simulink subsystem "Reefscape_Auto_sub"  (R2023b)
settings: Solver=VariableStepAuto  StartTime=0.0  StopTime=10.0  RelTol=1e-3
undefined symbols (not defined in the file): All_Paths_Num_Poses, All_Paths_Ref_Poses, AT_Steering_Error_Angle_Gain_P, AT_Steering_Speed_Max, AT_Translation_Control_Gain_Relative, AT_Translation_Speed_Max_Relative, Auto_Starting_Position
libraries: simulink x3
settings Model: Creator=ander  LastModifiedBy=ander

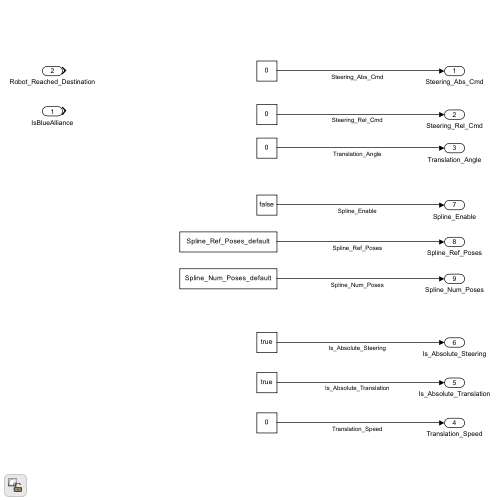
[thumbnail: Simulink's stored preview of the top-level diagram]
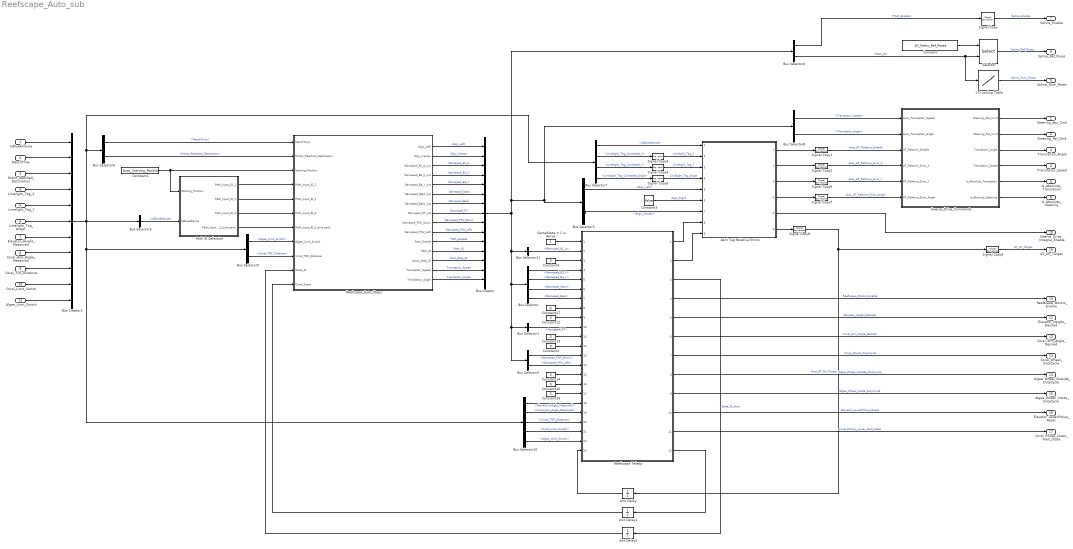
== system Reefscape_Auto_sub ==
  IsBlueAlliance : Inport
  MatchTime : Inport  Port=2
  Robot_Reached_Destination : Inport  Port=3
  Limelight_Tag_X : Inport  Port=4
  Limelight_Tag_Y : Inport  Port=5
  Limelight_Tag_Angle : Inport  Port=6
  Elevator_Height_Measured : Inport  Port=7
  Coral_Arm_Angle_Measured : Inport  Port=8
  Coral_TOF_Distance : Inport  Port=9
  Coral_Limit_Switch : Inport  Port=10
  Algae_Limit_Switch : Inport  Port=11
  1-D Lookup Table : Lookup_n-D  NumberOfTableDimensions=1  BreakpointsSpecification=Even spacing  BreakpointsForDimension1=[-5:5]  Table=All_Paths_Num_Poses  InterpMethod=Flat  InternalRulePriority=Speed  OutDataTypeStr=double  RndMeth=Simplest
  April Tag Relative Errors : Subsystem  ReferencedSubsystem=April_Tag_Relative_Errors
  Bus Creator : BusCreator  Inputs=15
  Bus Creator2 : BusCreator  Inputs=11
  Bus Selector : BusSelector  OutputSignals=Gamepad_B3_X,Gamepad_B4_Y,Gamepad_Start,Gamepad_Back
  Bus Selector1 : BusSelector  OutputSignals=Gamepad_RT
  Bus Selector10 : BusSelector  OutputSignals=Elevator_Height_Measured,Coral_Arm_Angle_Measured,Coral_TOF_Distance,Coral_Limit_Switch,Algae_Limit_Switch
  Bus Selector11 : BusSelector  OutputSignals=Gamepad_B1_A
  Bus Selector2 : BusSelector  OutputSignals=Gamepad_POV_Down,Gamepad_POV_Left
  Bus Selector3 : BusSelector  OutputSignals=Align_Left,Align_Center
  Bus Selector4 : BusSelector  OutputSignals=Path_Enable,Path_ID
  Bus Selector5 : BusSelector  OutputSignals=IsBlueAlliance
  Bus Selector6 : BusSelector  OutputSignals=MatchTime,Robot_Reached_Destination
  Bus Selector7 : BusSelector  OutputSignals=IsBlueAlliance,Limelight_Tag_Corrected_X,Limelight_Tag_Corrected_Y,Limelight_Tag_Corrected_Angle
  Bus Selector8 : BusSelector  OutputSignals=Translation_Speed,Translation_Angle
  Bus Selector9 : BusSelector  OutputSignals=Algae_Limit_Switch,Coral_TOF_Distance
  Constant : Constant  Value=All_Paths_Ref_Poses
  Constant1 : Constant  Value=Auto_Starting_Position  OutDataTypeStr=double
  Constant{2,4,12..14,17} (6 alike) : Constant  Value=0  OutDataTypeStr=boolean
  Constant15 : Constant  Value=0  OutDataTypeStr=double
  Constant16 : Constant  Value=0  OutDataTypeStr=double
  Constant3 : Constant  Value=false  OutDataTypeStr=boolean
  GameState = 1 is Autos : Constant  OutDataTypeStr=uint8
  Path ID Selection : Subsystem
  Reefscape Teleop : Subsystem  ReferencedSubsystem=Reefscape_Teleop_sub
  Reefscape_Auto_Steps : Stateflow chart  TreatAsAtomicUnit=on
      settings: PortSchema="{\"entries\":[{\"content\":{\"sides\":[{\"content\":{\"connectorIds\":[\"In1\",\"In2\",\"In3\",\"In4\",\"In5\",\"In6\",\"In7\",\"In8\",\"In9\",\"In11\",\"In10\"]},\"type\":\"ConnectorPlacement.EquallySpacedRectSide\",\"uuid\":\"b68629cc-4697-4054-9cba-8a9d44fa304a\"},{\"content\":{\"connectorIds\":[\"Out1\",\"Out2\",\"Out14\",\"Out15\",\"Out3\",\"Out4\",\"Out5\",\"Out6\",\"Out7\",\"Out8\",\"Out9\",\"Out10\",\"Out11\",\"Out12\",\"Out13\"],\"side\":\"RIGHT\"},\"type\":\"ConnectorPlacement.EquallySpacedRectSide\",\"uuid\":\"e5ec4660-532e-44af-95ac-1c70b52239a5\"},{\"content\":{\"side\":\"TOP\"},\"type\":\"ConnectorPlacement.EquallySpacedRectSide\",\"uuid\":\"c81c735c-b6d1-4ece-b5d5-793d4c0e4420\"}]},\"type\":\"ConnectorPlacement.EquallySpacedConnector\",\"uuid\":\"b2f2970a-f1c8-496a-85fd-16c79425c6c1\"}],\"packageUris\":[\"http://schema.mathworks.com/mf0/Connector/R2020b\"],\"version\":\"1.0\"}"
  Selector : Selector  NumberOfDimensions=3  InputPortWidth=3  IndexOptions=Select all,Select all,Index vector (port)  Indices=[1 3],1,1  OutputSizes=1,1,1
  Signal Copy{,1..9} (10 alike) : SignalConversion  OverrideOpt=off
  Swerve_Drive_Commands : Subsystem
  Unit Delay : UnitDelay  SampleTime=-1  HasFrameUpgradeWarning=on
  Unit Delay1 : UnitDelay  SampleTime=-1  HasFrameUpgradeWarning=on
  Unit Delay2 : UnitDelay  SampleTime=-1  HasFrameUpgradeWarning=on
  Steering_Abs_Cmd : Outport
  Steering_Rel_Cmd : Outport  Port=2
  Translation_Angle : Outport  Port=3
  Translation_Speed : Outport  Port=4
  Is_Absolute_Translation : Outport  Port=5
  Is_Absolute_Steering : Outport  Port=6
  Spline_Enable : Outport  Port=7
  Spline_Ref_Poses : Outport  Port=8
  Spline_Num_Poses : Outport  Port=9
  Reefscape_Motors_Enable : Outport  Port=10
  Elevator_Height_Desired : Outport  Port=11
  Coral_Arm_Angle_Desired : Outport  Port=12
  Coral_Wheel_DutyCycle : Outport  Port=13
  Algae_Wheel_Outside_DutyCycle : Outport  Port=14
  Algae_Wheel_Inside_DutyCycle : Outport  Port=15
  Elevator_LowerPickup_Reset : Outport  Port=16
  Coral_Pickup_Lower_Wait_State : Outport  Port=17
  Swerve_Drive_Integral_Enable : Outport  Port=18
  AT_On_Target : Outport  Port=19
  wires:
  Constant3/1 -> April Tag Relative Errors/6  "Align_Right"
  Unit Delay/1 -> Reefscape Teleop/23
  Bus Selector10/5 -> Reefscape Teleop/22  "<Algae_Limit_Switch>"
  Bus Selector10/4 -> Reefscape Teleop/21  "<Coral_Limit_Switch>"
  Bus Selector10/3 -> Reefscape Teleop/20  "<Coral_TOF_Distance>"
  Bus Selector10/2 -> Reefscape Teleop/19  "<Coral_Arm_Angle_Measured>"
  Bus Selector10/1 -> Reefscape Teleop/18  "<Elevator_Height_Measured>"
  Constant16/1 -> Reefscape Teleop/17
  Constant15/1 -> Reefscape Teleop/16
  Constant14/1 -> Reefscape Teleop/15
  Bus Selector2/2 -> Reefscape Teleop/14  "<Gamepad_POV_Left>"
  Bus Selector2/1 -> Reefscape Teleop/13  "<Gamepad_POV_Down>"
  Constant2/1 -> Reefscape Teleop/12
  1-D Lookup Table/1 -> Spline_Num_Poses/1  "Spline_Num_Poses"
  Signal Copy/1 -> Spline_Enable/1  "Spline_Enable"
  Selector/1 -> Spline_Ref_Poses/1  "Spline_Ref_Poses"
  Constant/1 -> Selector/1
  Bus Selector6/2 -> Reefscape_Auto_Steps/2(Robot_Reached_Destination)  "<Robot_Reached_Destination>"
  Constant1/1 -> Reefscape_Auto_Steps/3(Starting_Position), Path ID Selection/1(Starting_Position)
  Path ID Selection/3(Path_Input_ID_3) -> Reefscape_Auto_Steps/6(Path_Input_ID_3)
  Bus Selector5/1 -> Path ID Selection/2(IsBlueAlliance)  "<IsBlueAlliance>"
  Path ID Selection/1(Path_Input_ID_1) -> Reefscape_Auto_Steps/4(Path_Input_ID_1)
  Path ID Selection/2(Path_Input_ID_2) -> Reefscape_Auto_Steps/5(Path_Input_ID_2)
  Signal Copy5/1 -> April Tag Relative Errors/4  "Limelight_Tag_Angle"
  Signal Copy4/1 -> April Tag Relative Errors/3  "Limelight_Tag_Y"
  Signal Copy3/1 -> April Tag Relative Errors/2  "Limelight_Tag_X"
  Reefscape Teleop/1 -> April Tag Relative Errors/8
  Reefscape Teleop/2 -> April Tag Relative Errors/9
  April Tag Relative Errors/6 -> Signal Copy8/1
  Bus Creator/1 -> Bus Selector11/1, Bus Selector/1, Bus Selector1/1, Bus Selector2/1, Bus Selector4/1, Bus Selector8/1, Bus Selector3/1
  Bus Selector3/1 -> April Tag Relative Errors/5  "<Align_Left>"
  Bus Selector3/2 -> April Tag Relative Errors/7  "<Align_Center>"
  Reefscape_Auto_Steps/1(Align_Left) -> Bus Creator/1  "Align_Left"
  Reefscape_Auto_Steps/2(Align_Center) -> Bus Creator/2  "Align_Center"
  Unit Delay1/1 -> Reefscape_Auto_Steps/10(Coral_Score)
  Bus Selector4/1 -> Signal Copy/1  "<Path_Enable>"
  Bus Selector4/2 -> Selector/2, 1-D Lookup Table/1  "<Path_ID>"
  IsBlueAlliance/1 -> Bus Creator2/1
  Bus Creator2/1 -> Bus Selector10/1, Bus Selector9/1, Bus Selector5/1, Bus Selector6/1, Bus Selector7/1
  Bus Selector7/1 -> April Tag Relative Errors/1  "<IsBlueAlliance>"
  Bus Selector9/1 -> Reefscape_Auto_Steps/8(Algae_Limit_Switch)  "<Algae_Limit_Switch>"
  April Tag Relative Errors/2 -> Signal Copy2/1
  April Tag Relative Errors/1 -> Signal Copy1/1
  April Tag Relative Errors/3 -> Signal Copy6/1
  April Tag Relative Errors/4 -> Signal Copy7/1
  April Tag Relative Errors/5 -> Swerve_Drive_Integral_Enable/1
  Swerve_Drive_Commands/1(Steering_Abs_Cmd) -> Steering_Abs_Cmd/1
  Swerve_Drive_Commands/2(Steering_Rel_Cmd) -> Steering_Rel_Cmd/1
  Swerve_Drive_Commands/3(Translation_Angle) -> Translation_Angle/1
  Swerve_Drive_Commands/4(Translation_Speed) -> Translation_Speed/1
  Swerve_Drive_Commands/5(Is_Absolute_Translation) -> Is_Absolute_Translation/1
  Swerve_Drive_Commands/6(Is_Absolute_Steering) -> Is_Absolute_Steering/1
  Bus Selector8/2 -> Swerve_Drive_Commands/2(Auto_Translation_Angle)  "<Translation_Angle>"
  Bus Selector8/1 -> Swerve_Drive_Commands/1(Auto_Translation_Speed)  "<Translation_Speed>"
  Bus Selector7/2 -> Signal Copy3/1  "<Limelight_Tag_Corrected_X>"
  Bus Selector7/3 -> Signal Copy4/1  "<Limelight_Tag_Corrected_Y>"
  Bus Selector7/4 -> Signal Copy5/1  "<Limelight_Tag_Corrected_Angle>"
  Reefscape Teleop/4 -> Reefscape_Motors_Enable/1  "Reefscape_Motors_Enable"
  Reefscape Teleop/5 -> Elevator_Height_Desired/1  "Elevator_Height_Desired"
  Reefscape Teleop/6 -> Coral_Arm_Angle_Desired/1  "Coral_Arm_Angle_Desired"
  Reefscape Teleop/7 -> Coral_Wheel_DutyCycle/1  "Coral_Wheel_DutyCycle"
  Reefscape Teleop/8 -> Algae_Wheel_Outside_DutyCycle/1  "Algae_Wheel_Outside_DutyCycle"
  Reefscape Teleop/9 -> Algae_Wheel_Inside_DutyCycle/1  "Algae_Wheel_Inside_DutyCycle"
  Reefscape Teleop/10 -> Elevator_LowerPickup_Reset/1  "Elevator_LowerPickup_Reset"
  Reefscape Teleop/11 -> Coral_Pickup_Lower_Wait_State/1  "Coral_Pickup_Lower_Wait_State"
  GameState = 1 is Autos/1 -> Reefscape Teleop/1
  Reefscape Teleop/12 -> Unit Delay1/1
  Algae_Limit_Switch/1 -> Bus Creator2/11
  Coral_Limit_Switch/1 -> Bus Creator2/10
  Coral_TOF_Distance/1 -> Bus Creator2/9
  Coral_Arm_Angle_Measured/1 -> Bus Creator2/8
  Elevator_Height_Measured/1 -> Bus Creator2/7
  Limelight_Tag_Angle/1 -> Bus Creator2/6
  Limelight_Tag_Y/1 -> Bus Creator2/5
  Limelight_Tag_X/1 -> Bus Creator2/4
  Robot_Reached_Destination/1 -> Bus Creator2/3
  Signal Copy1/1 -> Swerve_Drive_Commands/3(AT_Relative_Enable)  "Auto_AT_Relative_Enable"
  Signal Copy2/1 -> Swerve_Drive_Commands/4(AT_Relative_Error_X)  "Auto_AT_Relative_Error_X"
  Signal Copy6/1 -> Swerve_Drive_Commands/5(AT_Relative_Error_Y)  "Auto_AT_Relative_Error_Y"
  Signal Copy7/1 -> Swerve_Drive_Commands/6(AT_Relative_Error_Angle)  "Auto_AT_Relative_Error_Angle"
  Signal Copy8/1 -> Unit Delay/1, Signal Copy9/1  "Auto_AT_On_Target"
  Signal Copy9/1 -> AT_On_Target/1  "AT_On_Target"
  Bus Selector9/2 -> Reefscape_Auto_Steps/9(Coral_TOF_Distance)  "<Coral_TOF_Distance>"
  Constant4/1 -> Reefscape Teleop/3
  Bus Selector/2 -> Reefscape Teleop/5  "<Gamepad_B4_Y>"
  Bus Selector/3 -> Reefscape Teleop/6  "<Gamepad_Start>"
  Bus Selector/4 -> Reefscape Teleop/7  "<Gamepad_Back>"
  Constant17/1 -> Reefscape Teleop/8
  Constant13/1 -> Reefscape Teleop/11
  Reefscape Teleop/3 -> Unit Delay2/1  "State_ID_Auto"
  Path ID Selection/4(Path_Input_ID_2_end_early) -> Reefscape_Auto_Steps/7(Path_Input_ID_2_end_early)
  Constant12/1 -> Reefscape Teleop/9
  Bus Selector1/1 -> Reefscape Teleop/10  "<Gamepad_RT>"
  Unit Delay2/1 -> Reefscape_Auto_Steps/11(State_ID)
  Reefscape_Auto_Steps/14(Gamepad_B1_A_out) -> Bus Creator/3  "Gamepad_B1_A"
  Reefscape_Auto_Steps/3(Gamepad_B4_Y_out) -> Bus Creator/5  "Gamepad_B4_Y"
  Reefscape_Auto_Steps/4(Gamepad_Start_out) -> Bus Creator/6  "Gamepad_Start"
  Reefscape_Auto_Steps/5(Gamepad_Back_out) -> Bus Creator/7  "Gamepad_Back"
  Reefscape_Auto_Steps/6(Gamepad_RT_out) -> Bus Creator/8  "Gamepad_RT"
  Reefscape_Auto_Steps/7(Gamepad_POV_Down) -> Bus Creator/9  "Gamepad_POV_Down"
  Reefscape_Auto_Steps/8(Gamepad_POV_Left) -> Bus Creator/10  "Gamepad_POV_Left"
  Reefscape_Auto_Steps/9(Path_Enable) -> Bus Creator/11  "Path_Enable"
  Reefscape_Auto_Steps/10(Path_ID) -> Bus Creator/12  "Path_ID"
  Reefscape_Auto_Steps/11(Autos_Step_ID) -> Bus Creator/13  "Auto_Step_ID"
  Reefscape_Auto_Steps/12(Translation_Speed) -> Bus Creator/14  "Translation_Speed"
  Reefscape_Auto_Steps/13(Translation_Angle) -> Bus Creator/15  "Translation_Angle"
  Bus Selector11/1 -> Reefscape Teleop/2  "<Gamepad_B1_A>"
  Reefscape_Auto_Steps/15(Gamepad_B3_X_out) -> Bus Creator/4  "Gamepad_B3_X"
  Bus Selector/1 -> Reefscape Teleop/4  "<Gamepad_B3_X>"
  MatchTime/1 -> Bus Creator2/2
  Bus Selector6/1 -> Reefscape_Auto_Steps/1(MatchTime)  "<MatchTime>"

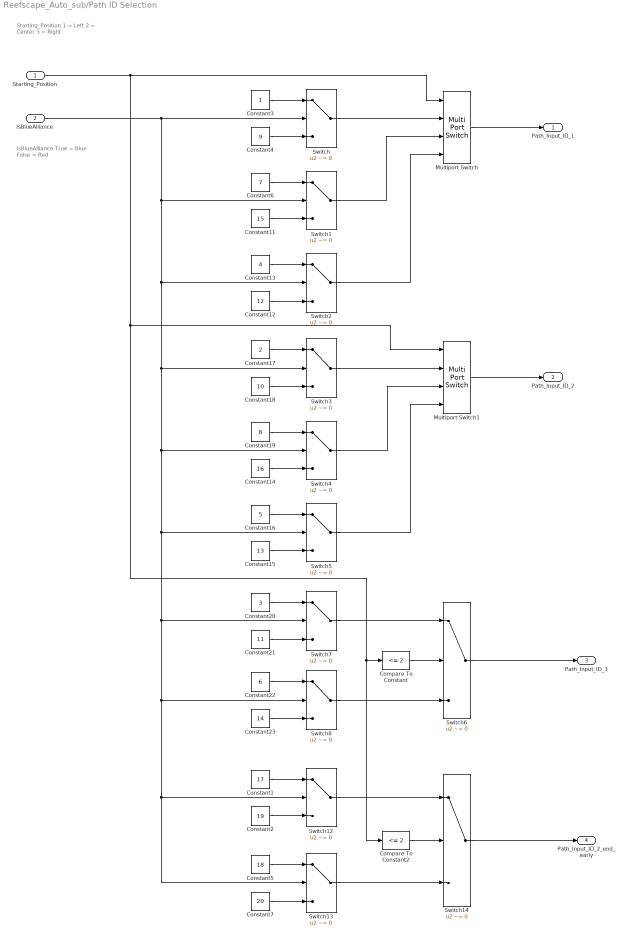
== system Reefscape_Auto_sub/Path ID Selection ==
  note: IsBlueAlliance
      | True = Blue
      | False = Red
  note: Starting_Position
      | 1 = Left
      | 2 = Center
      | 3 = Right
  Starting_Position : Inport
  IsBlueAlliance : Inport  Port=2
  Compare To Constant : simulink/Logic and Bit Operations/Compare To Constant  relop=<=  const=2  OutDataTypeStr=boolean
  Compare To Constant2 : simulink/Logic and Bit Operations/Compare To Constant  relop=<=  const=2  OutDataTypeStr=boolean
  Constant1 : Constant  Value=17  OutDataTypeStr=uint8
  Constant11 : Constant  Value=15  OutDataTypeStr=uint8
  Constant12 : Constant  Value=12  OutDataTypeStr=uint8
  Constant13 : Constant  Value=4  OutDataTypeStr=uint8
  Constant14 : Constant  Value=16  OutDataTypeStr=uint8
  Constant15 : Constant  Value=13  OutDataTypeStr=uint8
  Constant16 : Constant  Value=5  OutDataTypeStr=uint8
  Constant17 : Constant  Value=2  OutDataTypeStr=uint8
  Constant18 : Constant  Value=10  OutDataTypeStr=uint8
  Constant19 : Constant  Value=8  OutDataTypeStr=uint8
  Constant2 : Constant  Value=19  OutDataTypeStr=uint8
  Constant20 : Constant  Value=3  OutDataTypeStr=uint8
  Constant21 : Constant  Value=11  OutDataTypeStr=uint8
  Constant22 : Constant  Value=6  OutDataTypeStr=uint8
  Constant23 : Constant  Value=14  OutDataTypeStr=uint8
  Constant3 : Constant  OutDataTypeStr=uint8
  Constant4 : Constant  Value=9  OutDataTypeStr=uint8
  Constant5 : Constant  Value=18  OutDataTypeStr=uint8
  Constant6 : Constant  Value=7  OutDataTypeStr=uint8
  Constant7 : Constant  Value=20  OutDataTypeStr=uint8
  Multiport Switch : MultiPortSwitch  SaturateOnIntegerOverflow=off  InputSameDT=off
  Multiport Switch1 : MultiPortSwitch  SaturateOnIntegerOverflow=off  InputSameDT=off
  Switch{,1..8,12..14} (12 alike) : Switch  Criteria=u2 ~= 0  SaturateOnIntegerOverflow=off  InputSameDT=off
  Path_Input_ID_1 : Outport
  Path_Input_ID_2 : Outport  Port=2
  Path_Input_ID_3 : Outport  Port=3
  Path_Input_ID_2_end_early : Outport  Port=4
  wires:
  Switch14/1 -> Path_Input_ID_2_end_early/1
  IsBlueAlliance/1 -> Switch/2, Switch1/2, Switch2/2, Switch3/2, Switch4/2, Switch5/2, Switch7/2, Switch13/2, Switch12/2, Switch8/2
  Switch12/1 -> Switch14/1
  Switch13/1 -> Switch14/3
  Constant1/1 -> Switch12/1
  Compare To Constant2/1 -> Switch14/2
  Constant5/1 -> Switch13/1
  Constant2/1 -> Switch12/3
  Constant7/1 -> Switch13/3
  Switch6/1 -> Path_Input_ID_3/1
  Starting_Position/1 -> Multiport Switch1/1, Compare To Constant/1, Compare To Constant2/1, Multiport Switch/1
  Switch5/1 -> Multiport Switch1/4
  Constant22/1 -> Switch8/1
  Multiport Switch1/1 -> Path_Input_ID_2/1
  Constant13/1 -> Switch2/1
  Constant20/1 -> Switch7/1
  Multiport Switch/1 -> Path_Input_ID_1/1
  Constant19/1 -> Switch4/1
  Constant4/1 -> Switch/3
  Switch4/1 -> Multiport Switch1/3
  Switch8/1 -> Switch6/3
  Constant14/1 -> Switch4/3
  Constant12/1 -> Switch2/3
  Switch3/1 -> Multiport Switch1/2
  Compare To Constant/1 -> Switch6/2
  Switch7/1 -> Switch6/1
  Switch/1 -> Multiport Switch/2
  Constant11/1 -> Switch1/3
  Constant17/1 -> Switch3/1
  Switch1/1 -> Multiport Switch/3
  Constant15/1 -> Switch5/3
  Switch2/1 -> Multiport Switch/4
  Constant3/1 -> Switch/1
  Constant16/1 -> Switch5/1
  Constant21/1 -> Switch7/3
  Constant23/1 -> Switch8/3
  Constant6/1 -> Switch1/1
  Constant18/1 -> Switch3/3

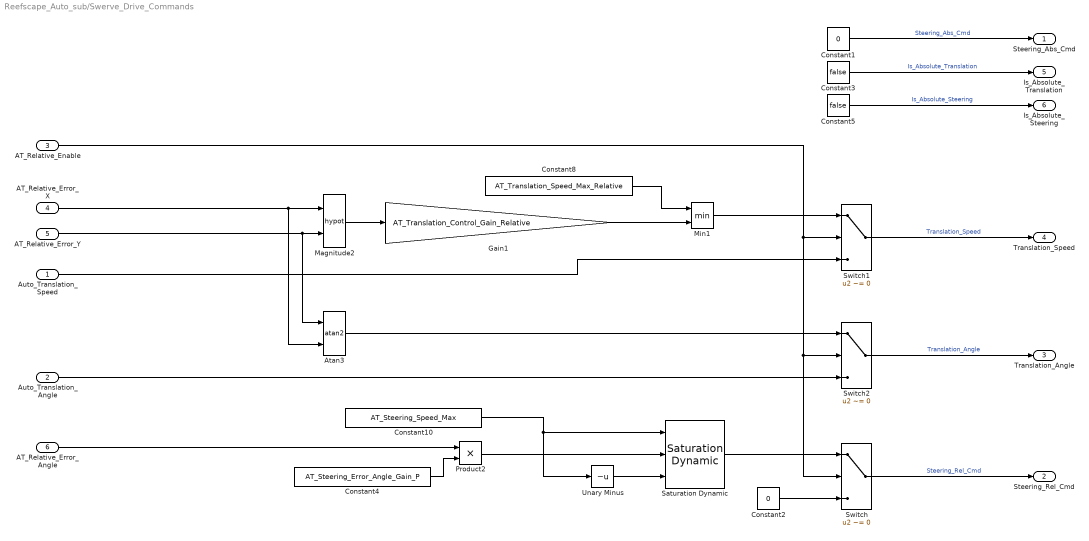
== system Reefscape_Auto_sub/Swerve_Drive_Commands ==
  Auto_Translation_Speed : Inport
  Auto_Translation_Angle : Inport  Port=2
  AT_Relative_Enable : Inport  Port=3
  AT_Relative_Error_X : Inport  Port=4
  AT_Relative_Error_Y : Inport  Port=5
  AT_Relative_Error_Angle : Inport  Port=6
  Atan3 : Trigonometry  Operator=atan2
  Constant1 : Constant  Value=0
  Constant10 : Constant  Value=AT_Steering_Speed_Max
  Constant2 : Constant  Value=0
  Constant3 : Constant  Value=false
  Constant4 : Constant  Value=AT_Steering_Error_Angle_Gain_P
  Constant5 : Constant  Value=false
  Constant8 : Constant  Value=AT_Translation_Speed_Max_Relative
  Gain1 : Gain  Gain=AT_Translation_Control_Gain_Relative
  Magnitude2 : Math  Operator=hypot
  Min1 : MinMax  Inputs=2
  Product2 : Product
  Saturation Dynamic : simulink/Discontinuities/Saturation Dynamic  OutMin=[]  OutMax=[]  OutDataTypeStr=Inherit: Same as second input  OutDataType=fixdt(1, 16)  OutScaling=2^-10  DoSatur=off
  Switch : Switch  Criteria=u2 ~= 0  SaturateOnIntegerOverflow=off  InputSameDT=off
  Switch1 : Switch  Criteria=u2 ~= 0  SaturateOnIntegerOverflow=off  InputSameDT=off
  Switch2 : Switch  Criteria=u2 ~= 0  SaturateOnIntegerOverflow=off  InputSameDT=off
  Unary Minus : UnaryMinus
  Steering_Abs_Cmd : Outport
  Steering_Rel_Cmd : Outport  Port=2
  Translation_Angle : Outport  Port=3
  Translation_Speed : Outport  Port=4
  Is_Absolute_Translation : Outport  Port=5
  Is_Absolute_Steering : Outport  Port=6
  wires:
  Auto_Translation_Angle/1 -> Switch2/3
  Auto_Translation_Speed/1 -> Switch1/3
  Constant2/1 -> Switch/3
  Constant3/1 -> Is_Absolute_Translation/1  "Is_Absolute_Translation"
  Constant1/1 -> Steering_Abs_Cmd/1  "Steering_Abs_Cmd"
  Constant5/1 -> Is_Absolute_Steering/1  "Is_Absolute_Steering"
  Switch1/1 -> Translation_Speed/1  "Translation_Speed"
  Switch2/1 -> Translation_Angle/1  "Translation_Angle"
  Switch/1 -> Steering_Rel_Cmd/1  "Steering_Rel_Cmd"
  Atan3/1 -> Switch2/1
  Min1/1 -> Switch1/1
  Product2/1 -> Saturation Dynamic/2
  AT_Relative_Enable/1 -> Switch1/2, Switch2/2, Switch/2
  Constant4/1 -> Product2/2
  AT_Relative_Error_Angle/1 -> Product2/1
  Constant10/1 -> Saturation Dynamic/1, Unary Minus/1
  Saturation Dynamic/1 -> Switch/1
  Unary Minus/1 -> Saturation Dynamic/3
  AT_Relative_Error_X/1 -> Atan3/2, Magnitude2/1
  Gain1/1 -> Min1/2
  Magnitude2/1 -> Gain1/1
  AT_Relative_Error_Y/1 -> Atan3/1, Magnitude2/2
  Constant8/1 -> Min1/1

== stateflow chart Reefscape_Auto_sub/Reefscape_Auto_Steps ==
  state Left_and_Right
    state Path_to_Reef_1
      en: Autos_Step_ID = 1;
      Translation_Speed = 0;
      Translation_Angle = 0;
      state Raise_to_L2
        en: Path_Enable = false;
        Gamepad_B3_X_out = true;
        timer = 0;
        du: timer = timer + 0.020;
        ex: Gamepad_B3_X_out = false;
      state Start
        en: Path_Enable = false;
        timer = 0;
        du: timer = timer + 0.020;
      state Drive
        en: Path_Enable = true;
        Path_ID = Path_Input_ID_1;
        state Stay_at_L2
          en: timer = 0;
          du: timer = timer + 0.020;
        state Raise_to_L4
          en: Gamepad_B4_Y_out = true;
          ex: Gamepad_B4_Y_out = false;
        (default) -> Stay_at_L2
        Stay_at_L2 -> Left_and_Right.Path_to_Reef_1.Drive.Raise_to_L4 : [timer >= Auto_Path1_Delay_to_L4_Time]
      (default) -> Left_and_Right.Path_to_Reef_1.Start
      Left_and_Right.Path_to_Reef_1.Start -> Raise_to_L2 : [timer >= 0.040]
      Raise_to_L2 -> Left_and_Right.Path_to_Reef_1.Drive : [timer >= Auto_Path1_Delay_to_L2_Time]
    state Score_at_Reef_1
      en: Autos_Step_ID = 2;
      Path_Enable = false;
      Translation_Speed = 0;
      Translation_Angle = 0;
      Align_Left = true;
      ex: Align_Left = false;
    state Back_Up_from_Reef_1
      en: Autos_Step_ID = 3;
      Path_Enable = false;
      Translation_Speed = Auto_Speed_Reef;
      Translation_Angle = pi;
      timer = 0;
      du: timer = timer + 0.020;
    state Path_to_Coral_Station_1
      en: Autos_Step_ID = 4;
      Path_Enable = true;
      Path_ID = Path_Input_ID_2;
      Translation_Speed = 0;
      Translation_Angle = 0;
      Gamepad_Start_out = true;
      ex: Gamepad_Start_out = false;
    state Path_to_Coral_Station_1_v3
      en: Autos_Step_ID = 20;
      Path_Enable = true;
      Path_ID = Path_Input_ID_2_end_early;
      Translation_Speed = 0;
      Translation_Angle = 0;
      Gamepad_Back_out = true;
      ex: Gamepad_Back_out = false;
    state Wait_at_Coral_Station_1
      en: Autos_Step_ID = 5;
      Path_Enable = false;
      Translation_Speed = Auto_Speed_Coral;
      Translation_Angle = pi;
    state Path_to_Reef_2
      en: Autos_Step_ID = 6;
      Path_Enable = true;
      Path_ID = Path_Input_ID_3;
      Translation_Speed = 0;
      Translation_Angle = 0;
      state Timer_to_L4
        en: timer = 0;
        du: timer = timer + 0.020;
      state Set_L4
        en: Gamepad_B4_Y_out = true;
        ex: Gamepad_B4_Y_out = false;
      (default) -> Timer_to_L4
      Timer_to_L4 -> Set_L4 : [timer >= Auto_Path2_Delay_to_L4_Time]
    state Path_to_Reef_2_v2
      en: Autos_Step_ID = 22;
      Path_Enable = true;
      Path_ID = Path_Input_ID_3;
      Translation_Speed = 0;
      Translation_Angle = 0;
      state L1
        en: Gamepad_B1_A_out = true;
        ex: Gamepad_B1_A_out = false;
      state Back
        en: Gamepad_Back_out = true;
        ex: Gamepad_Back_out = false;
      (default) -> L1
      L1 -> Left_and_Right.Path_to_Reef_2_v2.Back : [State_ID >= 2.1]
    state Score_at_Reef_2
      en: Autos_Step_ID = 7;
      Path_Enable = false;
      Translation_Speed = 0;
      Translation_Angle = 0;
      Align_Left = true;
      ex: Align_Left = false;
    state Back_Up_from_Reef_2
      en: Autos_Step_ID = 8;
      Path_Enable = false;
      Translation_Speed = Auto_Speed_Reef;
      Translation_Angle = pi;
      timer = 0;
      du: timer = timer + 0.020;
    state Back
      en: Gamepad_Back_out = true;
      ex: Gamepad_Back_out = false;
    state Wait_for_Teleop
      en: Autos_Step_ID = 15;
      Path_Enable = false;
      Translation_Speed = 0;
      Translation_Angle = 0;
    (default) -> Path_to_Reef_1
    Left_and_Right.Path_to_Reef_1.Drive -> Score_at_Reef_1 : [Robot_Reached_Destination]
    Score_at_Reef_1 -> Back_Up_from_Reef_1 : [Coral_Score]
    Back_Up_from_Reef_1 -> (junction 224) : [timer >= Auto_Backup_Time_Reef]
    (junction 224) -> (junction 154) [order 1] : [MatchTime <= MatchTime_Skip_Coral_Pickup]
    (junction 154) -> Path_to_Coral_Station_1_v3
    (junction 224) -> Path_to_Coral_Station_1 [order 2]
    Path_to_Coral_Station_1 -> Wait_at_Coral_Station_1 : [Robot_Reached_Destination]
    Path_to_Coral_Station_1_v3 -> (junction 158) : [Robot_Reached_Destination]
    Wait_at_Coral_Station_1 -> (junction 227) : [Coral_TOF_Distance < Coral_Detect_Distance]
    (junction 227) -> (junction 226) [order 1] : [MatchTime <= MatchTime_Skip_Second_L4]
    (junction 226) -> Path_to_Reef_2_v2
    (junction 227) -> Path_to_Reef_2 [order 2]
    Set_L4 -> Score_at_Reef_2 : [Robot_Reached_Destination]
    Left_and_Right.Path_to_Reef_2_v2.Back -> (junction 189) : [Robot_Reached_Destination]
    Score_at_Reef_2 -> Back_Up_from_Reef_2 : [Coral_Score]
    Back_Up_from_Reef_2 -> Left_and_Right.Back : [timer >= Auto_Backup_Time_Reef]
    Left_and_Right.Back -> Left_and_Right.Wait_for_Teleop
    (junction 189) -> Left_and_Right.Wait_for_Teleop
    (junction 158) -> (junction 189)
  state Center
    state Path_to_Reef
      en: Autos_Step_ID = 101;
      Translation_Speed = 0;
      Translation_Angle = 0;
      state Start
        en: Path_Enable = false;
        timer = 0;
        du: timer = timer + 0.020;
      state Raise_to_L4
        en:  Path_Enable = false;
        timer = 0;
        du: Gamepad_B4_Y_out = true;
        timer = timer + 0.020;
        ex: Gamepad_B4_Y_out = false;
      state Drive
        en:  Path_Enable = true;
        Path_ID = Path_Input_ID_1;
      (default) -> Center.Path_to_Reef.Start
      Center.Path_to_Reef.Start -> Center.Path_to_Reef.Raise_to_L4 : [timer >= 0.040]
      Center.Path_to_Reef.Raise_to_L4 -> Center.Path_to_Reef.Drive : [timer >= Auto_Path1_Delay_to_L4_Time]
    state Score_at_Reef
      en: Autos_Step_ID = 102;
      Path_Enable = false;
      Translation_Speed = 0;
      Translation_Angle = 0;
      Align_Left = true;
      ex: Align_Left = false;
    note: [Coral_Score]
    state Back_Up_from_Reef_Coral_Score
      en: Autos_Step_ID = 103;
      Path_Enable = false;
      Translation_Speed = Auto_Speed_Reef;
      Translation_Angle = pi;
      timer = 0;
      du: timer = timer + 0.020;
    state Adjust_Height_for_Algae
      en: Autos_Step_ID = 104;
      Path_Enable = false;
      Translation_Speed = 0;
      Translation_Angle = 0;
      Gamepad_POV_Left = true;
      timer = 0;
      du: timer = timer + 0.020;
      ex: Gamepad_POV_Left = false;
    state End_early
      en: Autos_Step_ID = 120;
      Path_Enable = false;
      Translation_Speed = 0;
      Translation_Angle = 0;
      Gamepad_Back_out = true;
      ex: Gamepad_Back_out = false;
    state Drive_Forward_and_Collect_Algae
      en: Autos_Step_ID = 105;
      Path_Enable = false;
      Translation_Speed = Auto_Speed_Algae;
      Translation_Angle = 0;
      Align_Center = true;
      ex: Align_Center = false;
    state Drive_Backward_from_Collect_Algae
      en: Autos_Step_ID = 106;
      Path_Enable = false;
      Translation_Speed = Auto_Speed_Reef;
      Translation_Angle = pi;
      timer = 0;
      du: timer = timer + 0.020;
    state Path_to_Processor
      en: Autos_Step_ID = 107;
      Path_Enable = true;
      Path_ID = Path_Input_ID_2;
      Gamepad_POV_Down = true;
      ex: Gamepad_POV_Down = false;
    state Score_at_Processor
      en: Autos_Step_ID = 108;
      Path_Enable = false;
      Translation_Speed = 0;
      Translation_Angle = 0;
      Gamepad_RT_out = true;
      ex: Gamepad_RT_out = false;
    state Drive_Backward_from_Processor
      en: Autos_Step_ID = 109;
      Path_Enable = false;
      Translation_Speed = Auto_Speed_Processor;
      Translation_Angle = pi;
      timer = 0;
      Gamepad_Back_out = true;
      du: timer = timer + 0.020;
      ex: Gamepad_Back_out = false;
    state Wait_for_Teleop
      en: Autos_Step_ID = 110;
      Path_Enable = false;
      Translation_Speed = 0;
      Translation_Angle = 0;
    (default) -> Path_to_Reef
    Center.Path_to_Reef.Drive -> Score_at_Reef : [Robot_Reached_Destination]
    Score_at_Reef -> Back_Up_from_Reef_Coral_Score : [Coral_Score]
    Back_Up_from_Reef_Coral_Score -> (junction 164) [order 2] : [false]
        | % [timer >= Auto_Backup_Time_Reef]
    (junction 164) -> End_early
    Back_Up_from_Reef_Coral_Score -> Adjust_Height_for_Algae [order 1] : [timer >= Auto_Backup_Time_Reef]
    Adjust_Height_for_Algae -> Drive_Forward_and_Collect_Algae : [timer >= Auto_Algae_Height_Time]
    End_early -> (junction 167)
    Drive_Forward_and_Collect_Algae -> Drive_Backward_from_Collect_Algae : [Algae_Limit_Switch]
    Drive_Backward_from_Collect_Algae -> Path_to_Processor : [timer >= Auto_Backup_Time_Reef]
    Path_to_Processor -> Score_at_Processor : [Robot_Reached_Destination]
    Score_at_Processor -> Drive_Backward_from_Processor : [~Algae_Limit_Switch]
    Drive_Backward_from_Processor -> Center.Wait_for_Teleop : [timer >= Auto_Backup_Time_Processor]
    (junction 167) -> Center.Wait_for_Teleop
  (default) -> (junction 52)
  (junction 52) -> Center [order 2]
  (junction 52) -> Left_and_Right [order 1] : % Left or Right
      | [Starting_Position == 1 || Starting_Position == 3]
  data: MatchTime input double; Align_Left output boolean =0; Align_Center output boolean =0; Gamepad_B4_Y_out output boolean =0; Gamepad_Start_out output boolean =0; Gamepad_Back_out output boolean =0; Gamepad_RT_out output boolean =0; Gamepad_POV_Down output boolean =0; Gamepad_POV_Left output boolean =0; Robot_Reached_Destination input boolean; Starting_Position input double; Path_Input_ID_1 input uint8; Path_Enable output boolean =0; Path_ID output uint8; timer local double =0; Path_Input_ID_2 input uint8; Path_Input_ID_3 input uint8; Path_Input_ID_2_end_early input uint8; Algae_Limit_Switch input boolean; Coral_TOF_Distance input double; Autos_Step_ID output uint8; Coral_Score input boolean; Auto_Speed_Coral parameter double; Auto_Speed_Algae parameter double; Auto_Speed_Reef parameter double; Auto_Backup_Time_Reef parameter double; Auto_Algae_Height_Time parameter double; Auto_Path2_Delay_to_L4_Time parameter double; Auto_Path1_Delay_to_L4_Time parameter double; Translation_Speed output double =0; Translation_Angle output double =0; Auto_Backup_Time_Processor parameter double; Auto_Speed_Processor parameter double; State_ID input double; Coral_Detect_Distance parameter double; Gamepad_B1_A_out output boolean =0; Auto_Path1_Delay_to_L2_Time parameter double; Gamepad_B3_X_out output boolean =0; MatchTime_Skip_Second_L4 parameter double; MatchTime_Skip_Coral_Pickup parameter double
